simulink model "position_2023b"  (R2023b)
settings: Solver=VariableStepAuto  StartTime=0.0  StopTime=1500  MaxStep=0.1  RelTol=1e-3  EnableMultiTasking=on
InitFcn:
  | % load parameters of the default quadrotor
  | disp('Quadrotor parameters loaded by InitFcn')
  | mdl_quadrotor
settings Model: Creator=corkep  LastModifiedBy=mejiasal
settings SolverCC: AlgebraicLoopSolver=TrustRegion  AutoInsertRateTranBlk=on
settings DataIOCC: LimitDataPoints=on  SaveFormat=Array  ReturnWorkspaceOutputs=off
settings OptimizationCC: BlockReduction=off  BooleanDataType=off  LifeSpan=inf
settings DebuggingCC: SaveWithParameterizedLinksMsg=none  MergeDetectMultiDrivingBlocksExec=none  SignalResolutionControl=TryResolveAllWithWarning  UnconnectedInputMsg=warning  UnconnectedOutputMsg=warning  UnconnectedLineMsg=warning  SFUnexpectedBacktrackingDiag=warning  SFNoUnconditionalDefaultTransitionDiag=warning  SFExecutionAtInitializationDiag=none  ArithmeticOperatorsInVariantConditions=warning
settings HardwareCC: ProdBitPerPointer=32  ProdBitPerSizeT=32  ProdBitPerPtrDiffT=32  ProdLargestAtomicFloat=None  ProdIntDivRoundTo=Undefined  ProdEndianess=Unspecified  ProdWordSize=32  ProdHWDeviceType=32-bit Generic  TargetUnknown=on
settings ModelReferenceCC: EnableRefExpFcnMdlSchedulingChecks=on  PropagateSignalLabelsOutOfModel=off
settings SFSimCC: SimUseLocalCustomCode=off  CustomCodeUndefinedFunction=UseInterfaceOnly
settings RTWCC: RTWUseLocalCustomCode=off
settings CodeAppCC: StateflowObjectComments=on
settings GRTTargetCC: TargetLangStandard=C89/C90 (ANSI)
settings ConfigComp: CovMetricSettings=dw  CovSaveCumulativeToWorkspaceVar=on  CovSaveSingleToWorkspaceVar=on  CovExternalEMLEnable=off  CovSFcnEnable=off

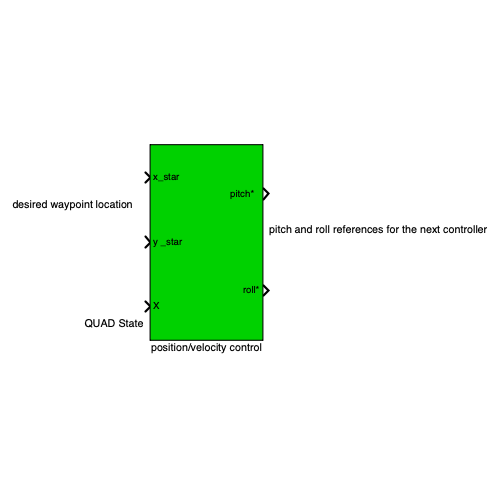
[thumbnail: Simulink's stored preview of the top-level diagram]
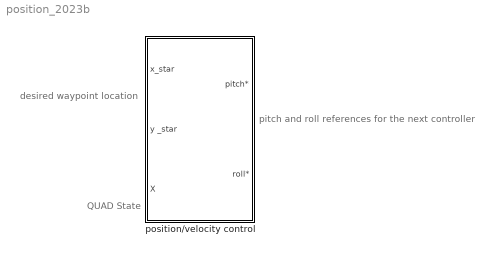
== system position_2023b ==
  note: pitch and roll references for the next controller
  note: desired waypoint location
  note: QUAD State
  position/velocity control : Subsystem

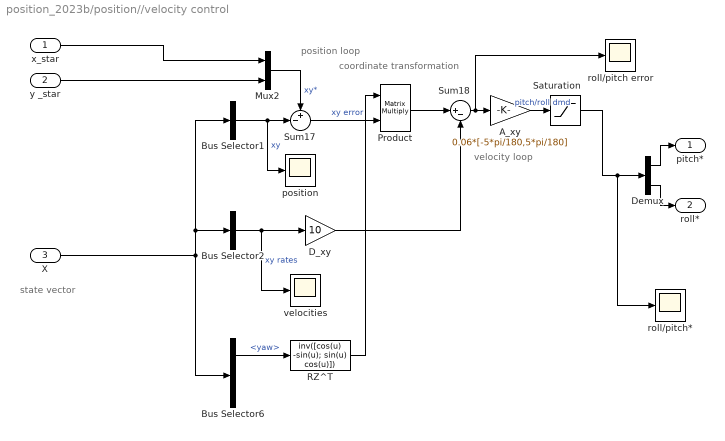
== system position_2023b/position//velocity control ==
  note: state vector
  note: position
      | loop
  note: velocity
      | loop
  note: coordinate transformation
  x_star : Inport
  y _star : Inport  Port=2
  X : Inport  Port=3
  A_xy : Gain  Gain=0.06*[-5*pi/180,5*pi/180]
  Bus Selector1 : BusSelector  OutputSignals=X,Y  OutputAsBus=on
  Bus Selector2 : BusSelector  OutputSignals=dx,dy  OutputAsBus=on
  Bus Selector6 : BusSelector  OutputSignals=yaw,dyaw
  D_xy : Gain  Gain=10
  Demux : Demux  Outputs=2
  Mux2 : Mux  Inputs=2
  Product : Product  Multiplication=Matrix(*)  RndMeth=Zero
  RZ^T : MATLABFcn  MATLABFcn=inv([cos(u) -sin(u); sin(u) cos(u)])  OutputDimensions=[2 2]  Output1D=off
  Saturation : Saturate  UpperLimit=0.35  LowerLimit=-0.35
  Sum17 : Sum  Inputs=+-|
  Sum18 : Sum  Inputs=|+-
  position : Scope
  roll/pitch error : Scope
  roll/pitch* : Scope
  velocities : Scope
  "pitch*  " : Outport  VectorParamsAs1DForOutWhenUnconnected=off
  roll* : Outport  Port=2  VectorParamsAs1DForOutWhenUnconnected=off
  wires:
  Demux/2 -> roll*/1
  Demux/1 -> "pitch*  "/1
  Product/1 -> Sum18/1
  D_xy/1 -> Sum18/2
  Sum18/1 -> roll/pitch error/1, A_xy/1
  Bus Selector6/1 -> RZ^T/1  "<yaw>"
  Sum17/1 -> Product/2  "xy error"
  Mux2/1 -> Sum17/1  "xy*"
  Bus Selector2/1 -> velocities/1, D_xy/1  "xy rates"
  RZ^T/1 -> Product/1
  Saturation/1 -> roll/pitch*/1, Demux/1
  X/1 -> Bus Selector6/1, Bus Selector1/1, Bus Selector2/1
  Bus Selector1/1 -> position/1, Sum17/2  "xy"
  x_star/1 -> Mux2/1
  y _star/1 -> Mux2/2
  A_xy/1 -> Saturation/1  "pitch/roll dmd"
